simulink model "chris_3R_hsv_mag"  (R2024b)
settings: Solver=FixedStepDiscrete  StartTime=0.0  StopTime=6  FixedStep=0.1  MaxStep=0.1  RelTol=1e-3
libraries: realtime_pacer_lib x1
(part 2 of 2)

== matlab function chris_3R_hsv_mag/Output_block_Robot_1/RGB to HSV to X,Y,th velocities/RGB to HSV ==
  data: R input; H output; G input; B input; S output; V output
function [H, S, V]= rgb2hsv_func(R, G, B)

% This one is tuned for the robot - pink

  % Clip RGB values to be within the range [100, 1200]
  R = max(min(R, 1800), 200);
  G = max(min(G, 2200), 250);
  B = max(min(B, 1900), 250);

  % Normalize RGB to [0, 1]
  R = (R - 200) / (1800-200); 
  G = (G - 250) / (2200-250);
  B = (B - 250) / (1900-250);

  Cmax = max(max(R, G), B);
  Cmin = min(min(R, G), B);
  delta = Cmax - Cmin;

  H = zeros(size(R));
  S = zeros(size(R));
  V = Cmax;

  % Calculate Hue
  ind = find(delta ~= 0); 
  r_ind = find((Cmax == R) & (delta ~= 0));
  g_ind = find((Cmax == G) & (delta ~= 0));
  b_ind = find((Cmax == B) & (delta ~= 0));

  H(r_ind) = 60 * mod((G(r_ind) - B(r_ind)) ./ delta(r_ind), 6);
  H(g_ind) = 60 * (((B(g_ind) - R(g_ind)) ./ delta(g_ind)) + 2);
  H(b_ind) = 60 * (((R(b_ind) - G(b_ind)) ./ delta(b_ind)) + 4);

  H = H / 360;

  % Calculate Saturation
  S(ind) = delta(ind) ./ Cmax(ind);

end

== matlab function chris_3R_hsv_mag/Output_block_Robot_1/RGB to HSV to X,Y,th velocities/S-Tuner ==
  data: h input; s_adjusted output; s input
function s_adjusted   = saturation_adjust(h,s)
    if 0 <= h && h <= 0.05
        s_adjusted = max(0, (s - 0.1114) * (0.7/0.9129) ) + 0.3;
    elseif 0.05 <= h && h <= 0.1
        s_adjusted = max(0, (s - 0.1915) * (0.7/0.665)) + 0.3;
    elseif 0.1 <= h && h <= 0.15
        s_adjusted = max(0, (s - 0.1613) * (0.7/0.6136)) + 0.3;
    elseif 0.15 <= h && h <= 0.2
        s_adjusted = max(0, (s - 0.1096) * (0.7/0.6058)) + 0.3;
    elseif 0.2 <= h && h <= 0.25
        s_adjusted = max(0, (s - 0.0677) * (0.7/0.5851)) + 0.3;
        
    elseif 0.25 <= h && h <= 0.3
        s_adjusted = max(0, (s + 0.1056) * (0.7/0.7955)) + 0.3;
    elseif 0.3 <= h && h <= 0.35
        s_adjusted = max(0, (s + 0.0671) * (0.7/0.644)) + 0.3;
    elseif 0.35 <= h && h <= 0.4
        s_adjusted = max(0, (s - 0.0036) * (0.7/0.3670)) + 0.3;
    elseif 0.4 <= h && h <= 0.45
        s_adjusted = max(0, (s - 0.0768) * (0.7/0.2182)) + 0.3;
    elseif 0.45 <= h && h <= 0.5
        s_adjusted = max(0, (s - 0.0453) * (0.7/0.4158)) + 0.3;

    elseif 0.5 <= h && h <= 0.55
        s_adjusted = max(0, (s - 0.0776) * (0.7/0.4708)) + 0.3;
    elseif 0.55 <= h && h <= 0.6
        s_adjusted = max(0, (s + 0.19) * (0.7/1.1235)) + 0.3;
    elseif 0.6 <= h && h <= 0.65
        s_adjusted = max(0, (s + 0.0663) * (0.7/0.9176)) + 0.3;
    elseif 0.65 <= h && h <= 0.7
        s_adjusted = max(0, (s - 0.0246) * (0.7/0.6231)) + 0.3;
    elseif 0.7 <= h && h <= 0.75
        s_adjusted = max(0, (s - 0.0774) * (0.7/0.5134)) + 0.3;       
        
    elseif 0.75 <= h && h <= 0.8
        s_adjusted = max(0, (s - 0.1307) * (0.7/0.4236)) + 0.3;
    elseif 0.8 <= h && h <= 0.85
        s_adjusted = max(0, (s - 0.2109) * (0.7/0.4814)) + 0.3;
    elseif 0.85 <= h && h <= 0.9
        s_adjusted = max(0, (s - 0.1347) * (0.7/0.7503)) + 0.3;
    elseif 0.9 <= h && h <= 0.95
        s_adjusted = max(0, (s - 0.0922) * (0.7/0.9583)) + 0.3;
    elseif 0.95 <= h && h <= 1
        s_adjusted = max(0, (s - 0.0796) * (0.7/1.0081)) + 0.3;
                
    else
        s_adjusted = s;  
    end
    
    s_adjusted = min(1, s_adjusted);
end

== matlab function chris_3R_hsv_mag/Output_block_Robot_1/RGB to HSV to X,Y,th velocities/hue-tuner ==
  data: h input; h_adjusted output
function h_adjusted   = hue_adjust(h)
    if 0.021 <= h && h <= 0.3
        h_adjusted = max(0, (h + 0.0207) * 1/0.739);
    elseif 0.3 <= h && h <= 0.5
        h_adjusted = max(0, (h + 0.5696) * 1/2.4058);
    elseif 0.5 <= h && h <= 0.7
        h_adjusted = max(0, h - 0.3632) * 1/0.4533 ;
    elseif 0.7 <= h && h <= .85
        h_adjusted = max(0, (h + 0.498) * 1/1.7413) ;
    elseif 0.85 <= h && h <= 1
        h_adjusted = max(0, (h - 0.6648) * 1/0.3342);
    else
        h_adjusted = h;
    end
    
    h_adjusted = min(1, h_adjusted);
end

== matlab function chris_3R_hsv_mag/Output_block_Robot_2/RGB to HSV to X,Y,th velocities/RGB to HSV ==
  data: R input; H output; G input; B input; S output; V output
function [H, S, V]= rgb2hsv_func(R, G, B)

% This one is tuned for the robot - pink

  % Clip RGB values to be within the range [100, 1200]
  R = max(min(R, 1800), 200);
  G = max(min(G, 2200), 250);
  B = max(min(B, 1900), 250);

  % Normalize RGB to [0, 1]
  R = (R - 200) / (1800-200); 
  G = (G - 250) / (2200-250);
  B = (B - 250) / (1900-250);

  Cmax = max(max(R, G), B);
  Cmin = min(min(R, G), B);
  delta = Cmax - Cmin;

  H = zeros(size(R));
  S = zeros(size(R));
  V = Cmax;

  % Calculate Hue
  ind = find(delta ~= 0); 
  r_ind = find((Cmax == R) & (delta ~= 0));
  g_ind = find((Cmax == G) & (delta ~= 0));
  b_ind = find((Cmax == B) & (delta ~= 0));

  H(r_ind) = 60 * mod((G(r_ind) - B(r_ind)) ./ delta(r_ind), 6);
  H(g_ind) = 60 * (((B(g_ind) - R(g_ind)) ./ delta(g_ind)) + 2);
  H(b_ind) = 60 * (((R(b_ind) - G(b_ind)) ./ delta(b_ind)) + 4);

  H = H / 360;

  % Calculate Saturation
  S(ind) = delta(ind) ./ Cmax(ind);

end

== matlab function chris_3R_hsv_mag/Output_block_Robot_2/RGB to HSV to X,Y,th velocities/S-Tuner ==
  data: h input; s_adjusted output; s input
function s_adjusted   = saturation_adjust(h,s)
    if 0 <= h && h <= 0.05
        s_adjusted = max(0, (s - 0.1114) * (0.7/0.9129) ) + 0.3;
    elseif 0.05 <= h && h <= 0.1
        s_adjusted = max(0, (s - 0.1915) * (0.7/0.665)) + 0.3;
    elseif 0.1 <= h && h <= 0.15
        s_adjusted = max(0, (s - 0.1613) * (0.7/0.6136)) + 0.3;
    elseif 0.15 <= h && h <= 0.2
        s_adjusted = max(0, (s - 0.1096) * (0.7/0.6058)) + 0.3;
    elseif 0.2 <= h && h <= 0.25
        s_adjusted = max(0, (s - 0.0677) * (0.7/0.5851)) + 0.3;
        
    elseif 0.25 <= h && h <= 0.3
        s_adjusted = max(0, (s + 0.1056) * (0.7/0.7955)) + 0.3;
    elseif 0.3 <= h && h <= 0.35
        s_adjusted = max(0, (s + 0.0671) * (0.7/0.644)) + 0.3;
    elseif 0.35 <= h && h <= 0.4
        s_adjusted = max(0, (s - 0.0036) * (0.7/0.3670)) + 0.3;
    elseif 0.4 <= h && h <= 0.45
        s_adjusted = max(0, (s - 0.0768) * (0.7/0.2182)) + 0.3;
    elseif 0.45 <= h && h <= 0.5
        s_adjusted = max(0, (s - 0.0453) * (0.7/0.4158)) + 0.3;

    elseif 0.5 <= h && h <= 0.55
        s_adjusted = max(0, (s - 0.0776) * (0.7/0.4708)) + 0.3;
    elseif 0.55 <= h && h <= 0.6
        s_adjusted = max(0, (s + 0.19) * (0.7/1.1235)) + 0.3;
    elseif 0.6 <= h && h <= 0.65
        s_adjusted = max(0, (s + 0.0663) * (0.7/0.9176)) + 0.3;
    elseif 0.65 <= h && h <= 0.7
        s_adjusted = max(0, (s - 0.0246) * (0.7/0.6231)) + 0.3;
    elseif 0.7 <= h && h <= 0.75
        s_adjusted = max(0, (s - 0.0774) * (0.7/0.5134)) + 0.3;       
        
    elseif 0.75 <= h && h <= 0.8
        s_adjusted = max(0, (s - 0.1307) * (0.7/0.4236)) + 0.3;
    elseif 0.8 <= h && h <= 0.85
        s_adjusted = max(0, (s - 0.2109) * (0.7/0.4814)) + 0.3;
    elseif 0.85 <= h && h <= 0.9
        s_adjusted = max(0, (s - 0.1347) * (0.7/0.7503)) + 0.3;
    elseif 0.9 <= h && h <= 0.95
        s_adjusted = max(0, (s - 0.0922) * (0.7/0.9583)) + 0.3;
    elseif 0.95 <= h && h <= 1
        s_adjusted = max(0, (s - 0.0796) * (0.7/1.0081)) + 0.3;
                
    else
        s_adjusted = s;  
    end
    
    s_adjusted = min(1, s_adjusted);
end

== matlab function chris_3R_hsv_mag/Output_block_Robot_2/RGB to HSV to X,Y,th velocities/hue-tuner ==
  data: h input; h_adjusted output
function h_adjusted   = hue_adjust(h)
    if 0.021 <= h && h <= 0.3
        h_adjusted = max(0, (h + 0.0207) * 1/0.739);
    elseif 0.3 <= h && h <= 0.5
        h_adjusted = max(0, (h + 0.5696) * 1/2.4058);
    elseif 0.5 <= h && h <= 0.7
        h_adjusted = max(0, h - 0.3632) * 1/0.4533 ;
    elseif 0.7 <= h && h <= .85
        h_adjusted = max(0, (h + 0.498) * 1/1.7413) ;
    elseif 0.85 <= h && h <= 1
        h_adjusted = max(0, (h - 0.6648) * 1/0.3342);
    else
        h_adjusted = h;
    end
    
    h_adjusted = min(1, h_adjusted);
end
